simulink model "Marx_Assignment_3 (2)"  (R2013a)
settings: Solver=ode23  SolverMode=SingleTasking  StartTime=0.0  StopTime=60e-6  RelTol=1e-3
libraries: powerlib x37
settings Model: CovHTMLOptions=-sRT=1 -aTS=1 -bRG=1 -bTC=1 -hTR=0 -nFC=0 -scm=1 -bcm=1 -xEv=0  CovSaveSingleToWorkspaceVar=off  Creator=ASUS  LastModifiedBy=SUJIT
settings DataIOCC: SignalLoggingSaveFormat=ModelDataLogs
settings OptimizationCC: BlockReduction=off  BooleanDataType=off
settings DebuggingCC: SaveWithParameterizedLinksMsg=none  SignalResolutionControl=TryResolveAllWithWarning  SolverPrmCheckMsg=none  MultiTaskDSMMsg=warning  MultiTaskCondExecSysMsg=none  StrictBusMsg=None
settings HardwareCC: TargetUnknown=on
settings RTWCC: IncludeERTFirstTime=on

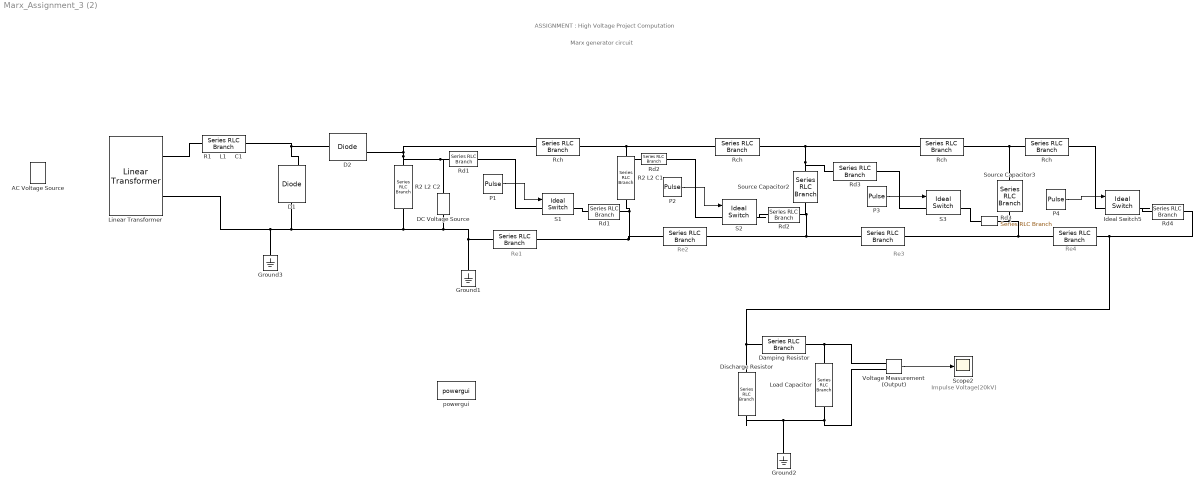
== system Marx_Assignment_3 (2) ==
  note: Impulse Voltage(20kV)
  note: Re1
  note: Re2
  note: Re3
  note: Re4
  note: Marx generator circuit
  note: ASSIGNMENT : High Voltage Project Computation
  "     " : powerlib/Elements/Series RLC Branch  LConnTagsString=__new0  RConnTagsString=__new0  BranchType=R  Resistance=1000  Inductance=1e-4  SetiL0=off  InitialCurrent=0  Capacitance=0  Setx0=off  InitialVoltage=0  Measurements=None
  "      " : powerlib/Elements/Series RLC Branch  LConnTagsString=__new0  RConnTagsString=__new0  BranchType=R  Resistance=1000  Inductance=1e-4  SetiL0=off  InitialCurrent=0  Capacitance=0  Setx0=off  InitialVoltage=0  Measurements=None
  "          " : powerlib/Elements/Series RLC Branch  LConnTagsString=__new0  RConnTagsString=__new0  BranchType=R  Resistance=750  Inductance=1e-4  SetiL0=off  InitialCurrent=0  Capacitance=0  Setx0=off  InitialVoltage=0  Measurements=None
  "                                                                  " : powerlib/Elements/Series RLC Branch  LConnTagsString=__new0  RConnTagsString=__new0  BranchType=R  Resistance=750  Inductance=1e-4  SetiL0=off  InitialCurrent=0  Capacitance=0  Setx0=off  InitialVoltage=0  Measurements=None
  "  Rd3  " : powerlib/Elements/Series RLC Branch  LConnTagsString=__new0  RConnTagsString=__new0  BranchType=R  Resistance=1e-5  Inductance=1e-5  SetiL0=off  InitialCurrent=0  Capacitance=1e-6  Setx0=off  InitialVoltage=0  Measurements=None
  " Rch" : powerlib/Elements/Series RLC Branch  LConnTagsString=__new0  RConnTagsString=__new0  BranchType=R  Resistance=750  Inductance=1e-5  SetiL0=off  InitialCurrent=0  Capacitance=1e-6  Setx0=off  InitialVoltage=0  Measurements=None
  AC Voltage Source : powerlib/Electrical Sources/AC Voltage Source  Amplitude=10000  Phase=0  Frequency=50  SampleTime=0  Measurements=None
  D1 : powerlib/Power Electronics/Diode  Ron=0.001  Lon=0  Vf=1  IC=0  UseSnubber=off  Rs=50000  Cs=250e-12  Measurements=on
  D2 : powerlib/Power Electronics/Diode  Ron=0.001  Lon=0  Vf=1  IC=0  UseSnubber=off  Rs=5000  Cs=250e-12  Measurements=on
  "DC Voltage Source " : powerlib/Electrical Sources/DC Voltage Source  Amplitude=5000  Measurements=None
  Damping Resistor : powerlib/Elements/Series RLC Branch  LConnTagsString=__new0  RConnTagsString=__new0  BranchType=R  Resistance=10/6  Inductance=1e-6  SetiL0=off  InitialCurrent=0  Capacitance=1e-7  Setx0=off  InitialVoltage=0  Measurements=None
  Discharge Resistor : powerlib/Elements/Series RLC Branch  LConnTagsString=__new0  RConnTagsString=__new0  BranchType=R  Resistance=1000  Inductance=1e-4  SetiL0=off  InitialCurrent=0  Capacitance=0  Setx0=off  InitialVoltage=0  Measurements=None
  Ground1 : powerlib/Elements/Ground  LConnTagsString=a
  Ground2 : powerlib/Elements/Ground  LConnTagsString=a
  Ground3 : powerlib/Elements/Ground  LConnTagsString=a
  Ideal Switch5 : powerlib/Power Electronics/Ideal Switch  Ron=0.0000000001  Lon=0  IC=0  Rs=1e10  Cs=inf  Measurements=on
  Linear Transformer : powerlib/Elements/Linear Transformer  LConnTagsString=a|b  RConnTagsString=A|B  UNITS=pu  NominalPower=[ 250e6 60 ]  winding1=[7.35e+05 0.002 0.08]  winding2=[7.35e+05 0.002 0.08]  ThreeWindings=off  winding3=[3.15e+05 0.002 0.08]  RmLm=[500.02 500]  Measurements=None  DataType=off
  Load Capacitor : powerlib/Elements/Series RLC Branch  LConnTagsString=__new0  RConnTagsString=__new0  BranchType=C  Resistance=0.00001  Inductance=1e-6  SetiL0=off  InitialCurrent=0  Capacitance=1e-7  Setx0=off  InitialVoltage=0  Measurements=None
  P1 : DiscretePulseGenerator  PulseType=Time based  Period=60e-6  PulseWidth=5
  P2 : DiscretePulseGenerator  PulseType=Time based  Period=1e-4
  P3 : DiscretePulseGenerator  PulseType=Time based  Period=1e-4
  P4 : DiscretePulseGenerator  PulseType=Time based  Period=1e-4
  R1     L1     C1 : powerlib/Elements/Series RLC Branch  LConnTagsString=__new0  RConnTagsString=__new0  BranchType=RLC  Resistance=1000  Inductance=0.001  SetiL0=off  InitialCurrent=0  Capacitance=1e-7  Setx0=off  InitialVoltage=0  Measurements=None
  R2 L2 C1 : powerlib/Elements/Series RLC Branch  LConnTagsString=__new0  RConnTagsString=__new0  BranchType=C  Resistance=100  Inductance=0.001  SetiL0=off  InitialCurrent=0  Capacitance=100e-6  Setx0=off  InitialVoltage=0  Measurements=Branch voltage
  R2 L2 C2 : powerlib/Elements/Series RLC Branch  LConnTagsString=__new0  RConnTagsString=__new0  BranchType=RLC  Resistance=1000  Inductance=0.001  SetiL0=off  InitialCurrent=0  Capacitance=1e-7  Setx0=off  InitialVoltage=0  Measurements=Branch voltage
  Rch : powerlib/Elements/Series RLC Branch  LConnTagsString=__new0  RConnTagsString=__new0  BranchType=R  Resistance=750  Inductance=1e-5  SetiL0=off  InitialCurrent=0  Capacitance=1e-6  Setx0=off  InitialVoltage=0  Measurements=None
  "Rch " : powerlib/Elements/Series RLC Branch  LConnTagsString=__new0  RConnTagsString=__new0  BranchType=R  Resistance=0.001  Inductance=1e-5  SetiL0=off  InitialCurrent=0  Capacitance=1e-6  Setx0=off  InitialVoltage=0  Measurements=None
  "Rch   " : powerlib/Elements/Series RLC Branch  LConnTagsString=__new0  RConnTagsString=__new0  BranchType=R  Resistance=750  Inductance=1e-5  SetiL0=off  InitialCurrent=0  Capacitance=1e-6  Setx0=off  InitialVoltage=0  Measurements=None
  Rd1 : powerlib/Elements/Series RLC Branch  LConnTagsString=__new0  RConnTagsString=__new0  BranchType=R  Resistance=1e-4  Inductance=1e-5  SetiL0=off  InitialCurrent=0  Capacitance=1e-6  Setx0=off  InitialVoltage=0  Measurements=None
  "Rd1  " : powerlib/Elements/Series RLC Branch  LConnTagsString=__new0  RConnTagsString=__new0  BranchType=R  Resistance=1e-5  Inductance=1e-5  SetiL0=off  InitialCurrent=0  Capacitance=1e-6  Setx0=off  InitialVoltage=0  Measurements=None
  Rd2 : powerlib/Elements/Series RLC Branch  LConnTagsString=__new0  RConnTagsString=__new0  BranchType=R  Resistance=1e-2  Inductance=1e-5  SetiL0=off  InitialCurrent=0  Capacitance=1e-6  Setx0=off  InitialVoltage=0  Measurements=None
  "Rd2  " : powerlib/Elements/Series RLC Branch  LConnTagsString=__new0  RConnTagsString=__new0  BranchType=R  Resistance=1e-5  Inductance=1e-5  SetiL0=off  InitialCurrent=0  Capacitance=1e-6  Setx0=off  InitialVoltage=0  Measurements=None
  "Rd3 " : powerlib/Elements/Series RLC Branch  LConnTagsString=__new0  RConnTagsString=__new0  BranchType=R  Resistance=1e-2  Inductance=1e-5  SetiL0=off  InitialCurrent=0  Capacitance=1e-6  Setx0=off  InitialVoltage=0  Measurements=None
  Rd4 : powerlib/Elements/Series RLC Branch  LConnTagsString=__new0  RConnTagsString=__new0  BranchType=R  Resistance=1e-5  Inductance=1e-5  SetiL0=off  InitialCurrent=0  Capacitance=1e-6  Setx0=off  InitialVoltage=0  Measurements=None
  S1 : powerlib/Power Electronics/Ideal Switch  Ron=0.0001  Lon=0  IC=0  Rs=1e10  Cs=inf  Measurements=on
  S2 : powerlib/Power Electronics/Ideal Switch  Ron=0.0000000001  Lon=0  IC=0  Rs=1e10  Cs=inf  Measurements=on
  S3 : powerlib/Power Electronics/Ideal Switch  Ron=0.0000000001  Lon=0  IC=0  Rs=1e10  Cs=inf  Measurements=on
  Scope2 : Scope
      settings: YMin=-0.004  YMax=0.006  SaveName=ScopeData4  MaxDataPoints=500000
  Source Capacitor2 : powerlib/Elements/Series RLC Branch  LConnTagsString=__new0  RConnTagsString=__new0  BranchType=C  Resistance=0.0001  Inductance=1  SetiL0=off  InitialCurrent=0  Capacitance=100e-6  Setx0=off  InitialVoltage=18000  Measurements=None
  Source Capacitor3 : powerlib/Elements/Series RLC Branch  LConnTagsString=__new0  RConnTagsString=__new0  BranchType=C  Resistance=0.0001  Inductance=1  SetiL0=off  InitialCurrent=0  Capacitance=100e-6  Setx0=off  InitialVoltage=18000  Measurements=None
  Voltage Measurement (Output) : powerlib/Measurements/Voltage Measurement  PhasorSimulation=off  OutputType=Complex  PSBequivalent=0
  powergui : powerlib/powergui  Priority=1  SimulationMode=Continuous  SolverType=Backward Euler  SampleTime=10e-7  frequency=60  SPID=off  DisableSnubberDevices=off  DisableRonSwitches=off  DisableVfSwitches=off  SwTol=0  Interpol=off  DisplayEquations=off  frequencyindice=0  Pbase=100e6  ErrMax=1e-4  Iterations=50  UnitsV=kV  UnitsW=MW  FunctionMessages=off  echomessages=off  HookPort=off  EnableUseOfTLC=off  x0status=blocks  RestoreLinks=warning  ResistiveCurrentMeasurement=off  Frange=[0:2:500]  Ylog=off  Xlog=on  ShowGrid=off  save=off  variable=ZData  ZoomFFT=off  StartTime=0.0  cycles=1  DisplayStyle=1  fundamental=60  FreqAxis=off  MaxFrequency=1000  frequencyindicesteady=1  RmsSteady=2  display=off  Ts=0  methode=off
  wires:
  P1/1 -> S1/1
  P2/1 -> S2/1
  P3/1 -> S3/1
  P4/1 -> Ideal Switch5/1
  Voltage Measurement (Output)/1 -> Scope2/1
  connections:
  Rd1/RConn1 -- S1/LConn1
  S1/RConn1 -- "Rd1  "/LConn1
  Rch/RConn1 -- Rd2/LConn1 -- R2 L2 C1/LConn1 -- "Rch   "/LConn1
  Rd2/RConn1 -- S2/LConn1
  S2/RConn1 -- "Rd2  "/LConn1
  "Rch   "/RConn1 -- "Rd3 "/LConn1 -- Source Capacitor2/LConn1 -- " Rch"/LConn1
  "Rd3 "/RConn1 -- S3/LConn1
  "Rch "/LConn1 -- Source Capacitor3/LConn1 -- " Rch"/RConn1
  "Rch "/RConn1 -- Ideal Switch5/LConn1
  Ideal Switch5/RConn1 -- Rd4/LConn1
  S3/RConn1 -- "  Rd3  "/LConn1
  Damping Resistor/LConn1 -- Rd4/RConn1 -- "      "/LConn1 -- Discharge Resistor/LConn1
  Load Capacitor/RConn1 -- Ground2/LConn1 -- Discharge Resistor/RConn1 -- Voltage Measurement (Output)/LConn2
  Damping Resistor/RConn1 -- Voltage Measurement (Output)/LConn1 -- Load Capacitor/LConn1
  "Rd1  "/RConn1 -- "                                                                  "/RConn1 -- "     "/LConn1 -- R2 L2 C1/RConn1
  Source Capacitor2/RConn1 -- "                                                                  "/LConn1 -- "          "/RConn1 -- "Rd2  "/RConn1
  "  Rd3  "/RConn1 -- "          "/LConn1 -- "      "/RConn1 -- Source Capacitor3/RConn1
  Linear Transformer/RConn2 -- D1/LConn1 -- "DC Voltage Source "/LConn1 -- "     "/RConn1 -- Ground1/LConn1 -- R2 L2 C2/RConn1 -- Ground3/LConn1
  D2/LConn1 -- R1     L1     C1/RConn1 -- D1/RConn1
  R1     L1     C1/LConn1 -- Linear Transformer/RConn1
  D2/RConn1 -- Rch/LConn1 -- "DC Voltage Source "/RConn1 -- Rd1/LConn1 -- R2 L2 C2/LConn1
